simulink model "imu_testing"  (R2014b)
settings: Solver=FixedStepDiscrete  StartTime=0.0  StopTime=inf  FixedStep=sample_time  RelTol=1e-3
StartFcn:
  | tg.sampletime = correctedSampleTime;
libraries: slrtlib x4
settings Model: SimulationMode=external  BufferReuse=off  Creator=wmartin  LastModifiedBy=drl
settings SolverCC: EnableConcurrentExecution=on
settings DataIOCC: LimitDataPoints=off  MaxDataPoints=1e7  SaveFormat=StructureWithTime  SignalLogging=off  DSMLogging=off
settings OptimizationCC: BlockReduction=off  OptimizeBlockIOStorage=off  BufferReuse=off  GlobalBufferReuse=off  ExpressionFolding=off  ExpressionDepthLimit=2147483647  LocalBlockOutputs=off  SimCompilerOptimization=On
settings DebuggingCC: UnderspecifiedInitializationDetection=Classic  MergeDetectMultiDrivingBlocksExec=none  StateNameClashWarn=warning
settings HardwareCC: ProdIntDivRoundTo=Zero  ProdEndianess=LittleEndian  ProdLongLongMode=on  ProdHWDeviceType=Generic->32-bit x86 compatible
settings ModelReferenceCC: UpdateModelReferenceTargets=IfOutOfDate  ModelReferenceNumInstancesAllowed=Single  ModelReferenceMinAlgLoopOccurrences=on
settings RTWCC: SystemTargetFile=slrt.tlc  TemplateMakefile=slrt_default_tmf  Description=Simulink Real-Time  RTWVerbose=off  ProcessScript=slrt_make_rtw_hook  RTWCompilerOptimization=On
settings CodeAppCC: MaxIdLength=256
settings SimulinkRealTimeCC: GeneratePreprocessorConditionals=Disable all  EnableShiftOperators=on  RL32LogBufSizeModifier=1e8

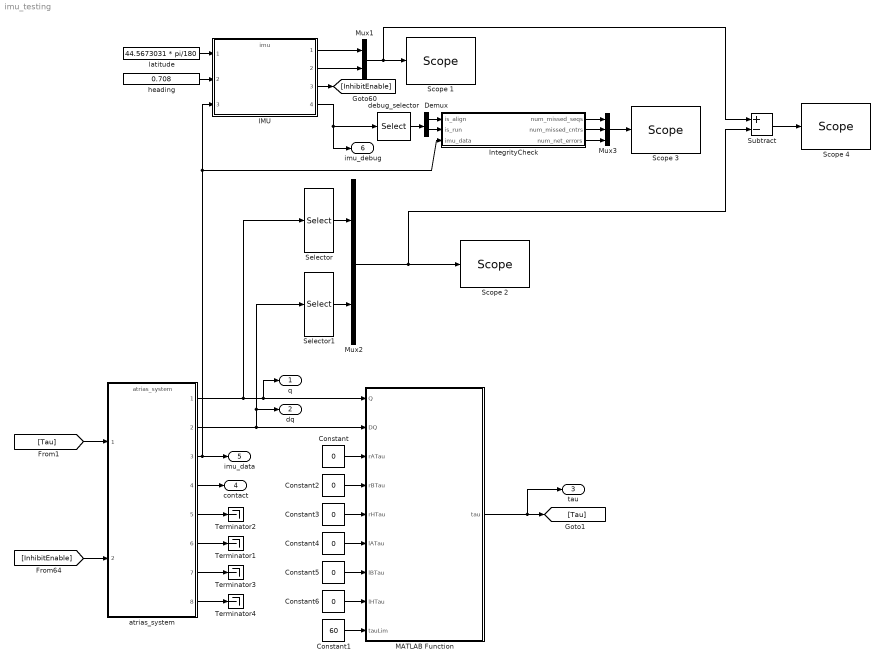
== system imu_testing ==
  Constant{,2..6} (6 alike) : Constant  Value=0
  Constant1 : Constant  Value=60
  Demux : Demux  Outputs=2
  IMU : ModelReference  ModelNameDialog=imu  SimulationMode=Normal  ModelReferenceVersion=1.2444  CopyOfModelName=imu  DefaultDataLogging=on
  IntegrityCheck : MATLAB Function  TreatAsAtomicUnit=on
  MATLAB Function : MATLAB Function  TreatAsAtomicUnit=on
  Mux1 : Mux  Inputs=2
  Mux2 : Mux  Inputs=2
  Mux3 : Mux  Inputs=3
  Scope 1 : slrtlib/Displays and Logging/Scope   scopeno=1  scopetype=Target  autostart=on  viewmode=Numerical  formatstr='%15.6f'  grid=on  ylimits=[0,0]  nosamples=10  noprepostsamples=0  interleave=1  triggermode=FreeRun  triggersignal=1  trigsignalfromport=off  triggerlevel=0.0  triggerslope=Either  triggerscope=1  triggersample=0  filename=data.dat  mode=Lazy  writesize=512  autorestart=off  dynamicfilemode=off  maxwritefilesize=512*1024^2
  Scope 2 : slrtlib/Displays and Logging/Scope   scopeno=6  scopetype=Target  autostart=on  viewmode=Numerical  formatstr='%15.6f'  grid=on  ylimits=[0,0]  nosamples=10  noprepostsamples=0  interleave=1  triggermode=FreeRun  triggersignal=1  trigsignalfromport=off  triggerlevel=0.0  triggerslope=Either  triggerscope=1  triggersample=0  filename=data.dat  mode=Lazy  writesize=512  autorestart=off  dynamicfilemode=off  maxwritefilesize=512*1024^2
  Scope 3 : slrtlib/Displays and Logging/Scope   scopeno=4  scopetype=Target  autostart=on  viewmode=Numerical  formatstr='%15.6f'  grid=on  ylimits=[0,0]  nosamples=10  noprepostsamples=0  interleave=1  triggermode=FreeRun  triggersignal=1  trigsignalfromport=off  triggerlevel=0.0  triggerslope=Either  triggerscope=1  triggersample=0  filename=data.dat  mode=Lazy  writesize=512  autorestart=off  dynamicfilemode=off  maxwritefilesize=512*1024^2
  Scope 4 : slrtlib/Displays and Logging/Scope   scopeno=2  scopetype=Target  autostart=on  viewmode=Numerical  formatstr='%15.6f'  grid=on  ylimits=[0,0]  nosamples=10  noprepostsamples=0  interleave=1  triggermode=FreeRun  triggersignal=1  trigsignalfromport=off  triggerlevel=0.0  triggerslope=Either  triggerscope=1  triggersample=0  filename=data.dat  mode=Lazy  writesize=512  autorestart=off  dynamicfilemode=off  maxwritefilesize=512*1024^2
  Selector : Selector  InputPortWidth=13  Indices=[11 12 13]
  Selector1 : Selector  InputPortWidth=13  Indices=[11 12 13]
  Subtract : Sum  Inputs=+-
  Terminator{1..4} (4 alike) : Terminator
  atrias_system : ModelReference  ModelNameDialog=atrias_system  SimulationMode=Normal  ModelReferenceVersion=1.2427  CopyOfModelName=atrias_system  DefaultDataLogging=on
  debug_selector : Selector  InputPortWidth=4  Indices=[3 4]
  heading : Constant  Value=0.708
  latitude : Constant  Value=44.5673031 * pi/180
  q : Outport
  dq : Outport  Port=2
  tau : Outport  Port=3
  contact : Outport  Port=4
  imu_data : Outport  Port=5
  imu_debug : Outport  Port=6
  wires:
  atrias_system/2 -> Selector1/1, dq/1, MATLAB Function/2(DQ)
  MATLAB Function/1(tau) -> [Tau], tau/1
  Constant/1 -> MATLAB Function/3(rATau)
  atrias_system/1 -> Selector/1, MATLAB Function/1(Q), q/1
  Constant1/1 -> MATLAB Function/9(tauLim)
  Constant3/1 -> MATLAB Function/5(rHTau)
  Constant2/1 -> MATLAB Function/4(rBTau)
  Constant4/1 -> MATLAB Function/6(lATau)
  Constant5/1 -> MATLAB Function/7(lBTau)
  Constant6/1 -> MATLAB Function/8(lHTau)
  atrias_system/4 -> contact/1
  atrias_system/6 -> Terminator1/1
  atrias_system/7 -> Terminator3/1
  atrias_system/5 -> Terminator2/1
  atrias_system/8 -> Terminator4/1
  atrias_system/3 -> imu_data/1, IMU/3, IntegrityCheck/3(imu_data)
  Selector/1 -> Mux2/1
  Selector1/1 -> Mux2/2
  IntegrityCheck/1(num_missed_seqs) -> Mux3/1
  Mux3/1 -> Scope 3/1
  IntegrityCheck/2(num_missed_cntrs) -> Mux3/2
  IntegrityCheck/3(num_net_errors) -> Mux3/3
  IMU/3 -> [InhibitEnable]
  [InhibitEnable] -> atrias_system/2
  [Tau] -> atrias_system/1
  latitude/1 -> IMU/1
  heading/1 -> IMU/2
  IMU/1 -> Mux1/1
  IMU/2 -> Mux1/2
  Mux1/1 -> Subtract/1, Scope 1/1
  IMU/4 -> debug_selector/1, imu_debug/1
  Demux/1 -> IntegrityCheck/1(is_align)
  Demux/2 -> IntegrityCheck/2(is_run)
  debug_selector/1 -> Demux/1
  Subtract/1 -> Scope 4/1
  Mux2/1 -> Scope 2/1, Subtract/2

== matlab function imu_testing/MATLAB Function ==
  data: Q input; tau output; DQ input; rATau input; rBTau input; rHTau input; lATau input; lBTau input; lHTau input; tauLim input
function tau  = torqueController(Q, DQ, rATau, rBTau, rHTau, lATau, lBTau, lHTau, tauLim)
%TRACKINGCONTROLLER Trajectory tracking contoller.
%
% Description:
%
% Notes:
% 	- State indexes (rBl rBm rAl rAm lBl lBm lAl lAm rHm lHm bR bY bP) 
%   - Input indexes (rB rA rH lB lA lH)
    
    % Output vector
    u = [rBTau rATau rHTau lBTau lATau lHTau];
    
    % Limit torques to be cautious
	tau = clamp(u, -tauLim, tauLim);

end % sampleController

function b = clamp(a, lim1, lim2)
%CLAMP Clamp value between two values.
	
	% Find which limit is min and max
	aMin = min(lim1);
	aMax = max(lim2);

	% Clamp value between limits
	b = max(min(a, aMax), aMin);
end % clamp

== matlab function imu_testing/IntegrityCheck ==
  data: is_align input; is_run input; imu_data input; num_missed_seqs output; num_missed_cntrs output; num_net_errors output
%function num_missed_seqs  = fcn(is_align, is_run, imu_data)
function [num_missed_seqs,num_missed_cntrs,num_net_errors] = fcn(is_align, is_run, imu_data)
%#codegen

persistent missed_seqs
persistent missed_cntrs
if isempty(missed_seqs)
    missed_seqs  = 0;
    missed_cntrs = zeros(numel(imu_data(9:end)), 1);
end

persistent prevSeq
persistent prevCntr
if isempty(prevSeq)
    prevSeq  = imu_data(7);
    prevCntr = imu_data(9:end);
end

persistent net_errors
if isempty(net_errors)
    net_errors = 0;
end

if logical(is_align) || logical(is_run)
    dseq  = mod(int16(imu_data(7)) - int16(prevSeq),  128);
    dcntr = mod(int16(imu_data(9:end)) - int16(prevCntr), 256);
    
    if dseq ~= 1
        missed_seqs = missed_seqs + 1;
    end
    
    %if dcntr ~= 1
    %    missed_cntrs = missed_cntrs + 1;
    %end
    missed_cntrs = missed_cntrs + double(dcntr ~= 1);
    
    net_errors = net_errors + sum(dcntr - 1);
end

prevSeq  = imu_data(7);
prevCntr = imu_data(9:end);

num_missed_seqs  = missed_seqs;
num_missed_cntrs = missed_cntrs;
num_net_errors   = net_errors;
